simulink model "GATE_B"  (R2016a)
settings: Solver=FixedStepDiscrete  StartTime=0.0  StopTime=10.0  FixedStep=0.001  RelTol=1e-3
values from neighbouring files (symbols this model uses):
  CLOSE_CHAR = CHAR_STAR    [GateParameter.m]
  CLOSE_SIDE_VALUE = single(4*ONE_SEC)    [GateParameter.m]
  CLOSED = uint8(12)    [GateParameter.m]
  CLOSING = uint8(13)    [GateParameter.m]
  CURRENT_STABLE_TIMER = uint8(200)    [GateParameter.m]
  CURRENT_THRESH = uint16(1000)    [GateParameter.m]
  INIT = uint8(15)    [GateParameter.m]
  MOVING_TIMER = uint32(60*ONE_SEC)    [GateParameter.m]
  NO_PASS_ASSIG = uint8(6)    [GateParameter.m]
  OPEN = uint8(14)    [GateParameter.m]
  OPEN_CHAR = CHAR_HASH    [GateParameter.m]
  OPEN_SIDE_VALUE = uint16(4*ONE_SEC)    [GateParameter.m]
  OPENING = uint8(11)    [GateParameter.m]
  OPENING_ACTIVE = uint8(1)    [GateParameter.m]
  PASS_ASSIGNED = uint8(7)    [GateParameter.m]
  PASS_INCOMPLETE = uint8(8)    [GateParameter.m]
  PASS_TIMEOUT = uint16(10*ONE_SEC)    [GateParameter.m]
  PASSWORD_VERIFIED = uint8(5)    [GateParameter.m]
  STABLE_TIMER_VALUE = uint16(1*ONE_SEC)    [GateParameter.m]
  TIMEOUT = uint8(9)    [GateParameter.m]
  WRONG_PASSWORD = uint8(2)    [GateParameter.m]
settings Model: ExtModeTrigDuration=2  Creator=omaro  LastModifiedBy=oelkawok
settings OptimizationCC: DefaultParameterBehavior=Inlined  OptimizeModelRefInitCode=on  LifeSpan=1
settings HardwareCC: ProdLongLongMode=on
settings RTWCC: SystemTargetFile=ert.tlc  TemplateMakefile=ert_default_tmf  GenerateReport=on  IncludeHyperlinkInReport=on  LaunchReport=on  PortableWordSizes=on  GenerateTraceInfo=on  GenerateTraceReport=on  GenerateTraceReportSl=on  GenerateTraceReportSf=on  GenerateTraceReportEml=on
settings CodeAppCC: ForceParamTrailComments=on  IgnoreCustomStorageClasses=off  OperatorAnnotations=on  SimulinkDataObjDesc=on  SFDataObjDesc=on  MATLABFcnDesc=on  InsertBlockDesc=on  MATLABSourceComments=on
settings ERTTargetCC: GenerateSampleERTMain=on  InlinedParameterPlacement=NonHierarchical  ERTCustomFileTemplate=example_file_process.tlc

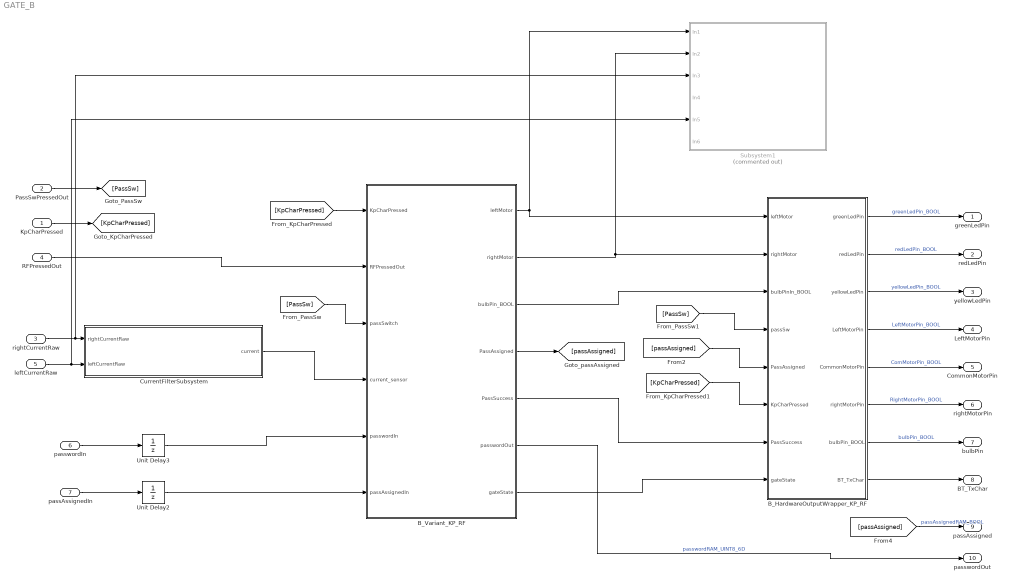
== system GATE_B ==
  KpCharPressed : Inport  OutDataTypeStr=uint8
  PassSwPressedOut : Inport  Port=2  OutDataTypeStr=boolean
  rightCurrentRaw : Inport  Port=3  OutDataTypeStr=uint16
  RFPressedOut : Inport  Port=4  OutDataTypeStr=uint8
  leftCurrentRaw : Inport  Port=5  OutDataTypeStr=uint16
  passwordIn : Inport  Port=6  OutDataTypeStr=uint8  PortDimensions=6
  passAssignedIn : Inport  Port=7  OutDataTypeStr=boolean
  B_HardwareOutputWrapper_KP_RF : Subsystem  VariantControl=Variant2
  B_Variant_KP_RF : Subsystem  VariantControl=Variant2
  CurrentFilterSubsystem : Subsystem
  Subsystem1 : Subsystem  Commented=on
  Unit Delay2 : UnitDelay  SampleTime=-1
  Unit Delay3 : UnitDelay  SampleTime=-1
  greenLedPin : Outport  OutDataTypeStr=boolean  PortDimensions=1  SampleTime=[0.001,0]
  redLedPin : Outport  Port=2  OutDataTypeStr=boolean  PortDimensions=1  SampleTime=[0.001,0]
  yellowLedPin : Outport  Port=3  OutDataTypeStr=boolean  PortDimensions=1  SampleTime=[0.001,0]
  LeftMotorPin : Outport  Port=4  OutDataTypeStr=boolean  PortDimensions=1  SampleTime=[0.001,0]
  CommonMotorPin : Outport  Port=5  OutDataTypeStr=boolean  PortDimensions=1  SampleTime=[0.001,0]
  rightMotorPin : Outport  Port=6  OutDataTypeStr=boolean  PortDimensions=1  SampleTime=[0.001,0]
  bulbPin : Outport  Port=7  OutDataTypeStr=boolean  PortDimensions=1  SampleTime=[0.001,0]
  BT_TxChar : Outport  Port=8  OutDataTypeStr=double  PortDimensions=1  SampleTime=[0.001,0]
  passAssigned : Outport  Port=9  OutDataTypeStr=boolean  PortDimensions=1  SampleTime=[0.001,0]
  passwordOut : Outport  Port=10  OutDataTypeStr=uint8  PortDimensions=6  SampleTime=[0.001,0]
  wires:
  CurrentFilterSubsystem/1(current) -> B_Variant_KP_RF/4(current_sensor)
  B_Variant_KP_RF/5(PassSuccess) -> B_HardwareOutputWrapper_KP_RF/7(PassSuccess)
  Unit Delay3/1 -> B_Variant_KP_RF/5(passwordIn)
  Unit Delay2/1 -> B_Variant_KP_RF/6(passAssignedIn)
  B_Variant_KP_RF/6(passwordOut) -> passwordOut/1  "passwordRAM_UINT8_6D"
  [passAssigned] -> B_HardwareOutputWrapper_KP_RF/5(PassAssigned)
  B_Variant_KP_RF/4(PassAssigned) -> [passAssigned]
  B_HardwareOutputWrapper_KP_RF/8(BT_TxChar) -> BT_TxChar/1
  B_HardwareOutputWrapper_KP_RF/7(bulbPin_BOOL) -> bulbPin/1  "bulbPin_BOOL"
  B_HardwareOutputWrapper_KP_RF/6(rightMotorPin) -> rightMotorPin/1  "RightMotorPin_BOOL"
  B_HardwareOutputWrapper_KP_RF/5(CommonMotorPin) -> CommonMotorPin/1  "ComMotorPin_BOOL"
  B_HardwareOutputWrapper_KP_RF/4(LeftMotorPin) -> LeftMotorPin/1  "LeftMotorPin_BOOL"
  B_HardwareOutputWrapper_KP_RF/3(yellowLedPin) -> yellowLedPin/1  "yellowLedPin_BOOL"
  B_HardwareOutputWrapper_KP_RF/2(redLedPin) -> redLedPin/1  "redLedPin_BOOL"
  B_HardwareOutputWrapper_KP_RF/1(greenLedPin) -> greenLedPin/1  "greenLedPin_BOOL"
  [KpCharPressed] -> B_HardwareOutputWrapper_KP_RF/6(KpCharPressed)
  [PassSw] -> B_HardwareOutputWrapper_KP_RF/4(passSw)
  B_Variant_KP_RF/3(bulbPin_BOOL) -> B_HardwareOutputWrapper_KP_RF/3(bulbPinIn_BOOL)
  B_Variant_KP_RF/1(leftMotor) -> B_HardwareOutputWrapper_KP_RF/1(leftMotor), Subsystem1/1(In1)
  [KpCharPressed] -> B_Variant_KP_RF/1(KpCharPressed)
  rightCurrentRaw/1 -> CurrentFilterSubsystem/1(rightCurrentRaw), Subsystem1/3(In3)
  [PassSw] -> B_Variant_KP_RF/3(passSwitch)
  RFPressedOut/1 -> B_Variant_KP_RF/2(RFPressedOut)
  KpCharPressed/1 -> [KpCharPressed]
  PassSwPressedOut/1 -> [PassSw]
  leftCurrentRaw/1 -> CurrentFilterSubsystem/2(leftCurrentRaw), Subsystem1/5(In5)
  [passAssigned] -> passAssigned/1  "passAssignedRAM_BOOL"
  passAssignedIn/1 -> Unit Delay2/1
  passwordIn/1 -> Unit Delay3/1
  B_Variant_KP_RF/2(rightMotor) -> B_HardwareOutputWrapper_KP_RF/2(rightMotor), Subsystem1/2(In2)
  B_Variant_KP_RF/7(gateState) -> B_HardwareOutputWrapper_KP_RF/8(gateState)

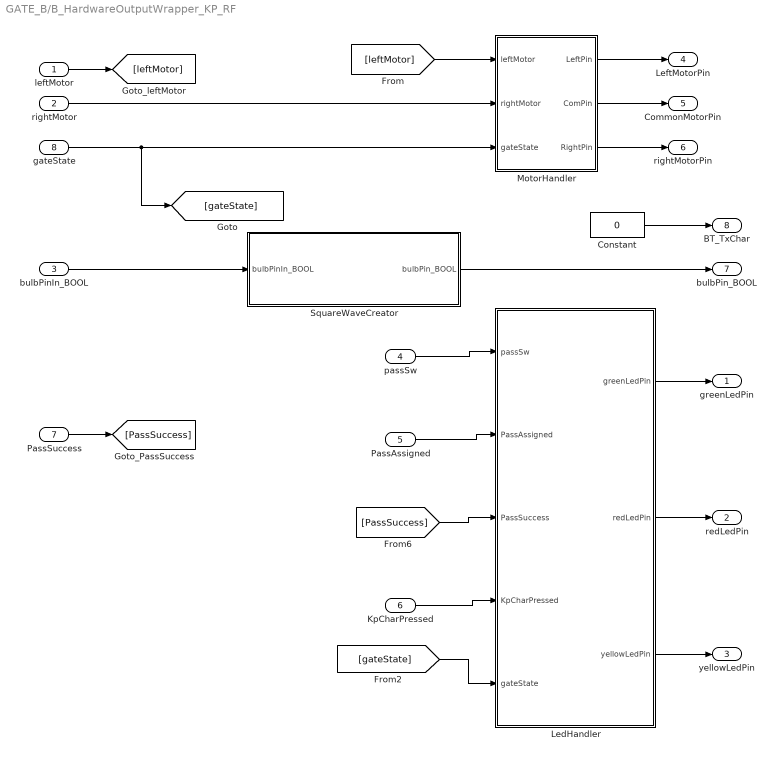
== system GATE_B/B_HardwareOutputWrapper_KP_RF ==
  leftMotor : Inport
  rightMotor : Inport  Port=2
  bulbPinIn_BOOL : Inport  Port=3
  passSw : Inport  Port=4
  PassAssigned : Inport  Port=5
  KpCharPressed : Inport  Port=6
  PassSuccess : Inport  Port=7
  gateState : Inport  Port=8
  Constant : Constant  Value=0  SampleTime=-1
  LedHandler : Subsystem
  MotorHandler : Subsystem
  SquareWaveCreator : Subsystem
  greenLedPin : Outport
  redLedPin : Outport  Port=2
  yellowLedPin : Outport  Port=3
  LeftMotorPin : Outport  Port=4
  CommonMotorPin : Outport  Port=5
  rightMotorPin : Outport  Port=6
  bulbPin_BOOL : Outport  Port=7
  BT_TxChar : Outport  Port=8
  wires:
  [gateState] -> LedHandler/5(gateState)
  SquareWaveCreator/1(bulbPin_BOOL) -> bulbPin_BOOL/1
  gateState/1 -> MotorHandler/3(gateState), [gateState]
  Constant/1 -> BT_TxChar/1
  PassSuccess/1 -> [PassSuccess]
  KpCharPressed/1 -> LedHandler/4(KpCharPressed)
  [PassSuccess] -> LedHandler/3(PassSuccess)
  PassAssigned/1 -> LedHandler/2(PassAssigned)
  passSw/1 -> LedHandler/1(passSw)
  leftMotor/1 -> [leftMotor]
  bulbPinIn_BOOL/1 -> SquareWaveCreator/1(bulbPinIn_BOOL)
  MotorHandler/3(RightPin) -> rightMotorPin/1
  MotorHandler/2(ComPin) -> CommonMotorPin/1
  MotorHandler/1(LeftPin) -> LeftMotorPin/1
  LedHandler/3(yellowLedPin) -> yellowLedPin/1
  LedHandler/2(redLedPin) -> redLedPin/1
  LedHandler/1(greenLedPin) -> greenLedPin/1
  [leftMotor] -> MotorHandler/1(leftMotor)
  rightMotor/1 -> MotorHandler/2(rightMotor)

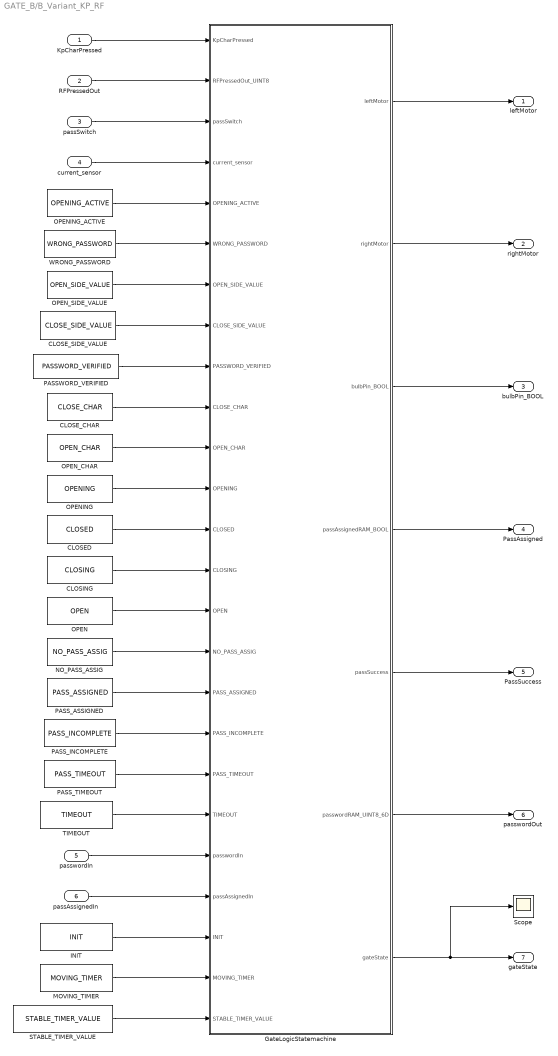
== system GATE_B/B_Variant_KP_RF ==
  KpCharPressed : Inport
  RFPressedOut : Inport  Port=2
  passSwitch : Inport  Port=3
  current_sensor : Inport  Port=4
  passwordIn : Inport  Port=5
  passAssignedIn : Inport  Port=6
  CLOSED : Constant  Value=CLOSED  SampleTime=-1
  CLOSE_CHAR : Constant  Value=CLOSE_CHAR  SampleTime=-1
  CLOSE_SIDE_VALUE : Constant  Value=CLOSE_SIDE_VALUE  SampleTime=-1
  CLOSING : Constant  Value=CLOSING  SampleTime=-1
  GateLogicStatemachine : Stateflow chart  TreatAsAtomicUnit=on
  INIT : Constant  Value=INIT  SampleTime=-1
  MOVING_TIMER : Constant  Value=MOVING_TIMER  SampleTime=-1
  NO_PASS_ASSIG : Constant  Value=NO_PASS_ASSIG  SampleTime=-1
  OPEN : Constant  Value=OPEN  SampleTime=-1
  OPENING : Constant  Value=OPENING  SampleTime=-1
  OPENING_ACTIVE : Constant  Value=OPENING_ACTIVE  SampleTime=-1
  OPEN_CHAR : Constant  Value=OPEN_CHAR  SampleTime=-1
  OPEN_SIDE_VALUE : Constant  Value=OPEN_SIDE_VALUE  SampleTime=-1
  PASSWORD_VERIFIED : Constant  Value=PASSWORD_VERIFIED  SampleTime=-1
  PASS_ASSIGNED : Constant  Value=PASS_ASSIGNED  SampleTime=-1
  PASS_INCOMPLETE : Constant  Value=PASS_INCOMPLETE  SampleTime=-1
  PASS_TIMEOUT : Constant  Value=PASS_TIMEOUT  SampleTime=-1
  STABLE_TIMER_VALUE : Constant  Value=STABLE_TIMER_VALUE  SampleTime=-1
  Scope : Scope
  TIMEOUT : Constant  Value=TIMEOUT  SampleTime=-1
  WRONG_PASSWORD : Constant  Value=WRONG_PASSWORD  SampleTime=-1
  leftMotor : Outport
  rightMotor : Outport  Port=2
  bulbPin_BOOL : Outport  Port=3
  PassAssigned : Outport  Port=4
  PassSuccess : Outport  Port=5
  passwordOut : Outport  Port=6
  gateState : Outport  Port=7
  wires:
  STABLE_TIMER_VALUE/1 -> GateLogicStatemachine/25(STABLE_TIMER_VALUE)
  MOVING_TIMER/1 -> GateLogicStatemachine/24(MOVING_TIMER)
  INIT/1 -> GateLogicStatemachine/23(INIT)
  GateLogicStatemachine/7(gateState) -> gateState/1, Scope/1
  CLOSING/1 -> GateLogicStatemachine/14(CLOSING)
  OPENING/1 -> GateLogicStatemachine/12(OPENING)
  CLOSED/1 -> GateLogicStatemachine/13(CLOSED)
  OPEN_CHAR/1 -> GateLogicStatemachine/11(OPEN_CHAR)
  CLOSE_CHAR/1 -> GateLogicStatemachine/10(CLOSE_CHAR)
  OPEN/1 -> GateLogicStatemachine/15(OPEN)
  PASSWORD_VERIFIED/1 -> GateLogicStatemachine/9(PASSWORD_VERIFIED)
  RFPressedOut/1 -> GateLogicStatemachine/2(RFPressedOut_UINT8)
  GateLogicStatemachine/3(bulbPin_BOOL) -> bulbPin_BOOL/1
  current_sensor/1 -> GateLogicStatemachine/4(current_sensor)
  WRONG_PASSWORD/1 -> GateLogicStatemachine/6(WRONG_PASSWORD)
  GateLogicStatemachine/1(leftMotor) -> leftMotor/1
  GateLogicStatemachine/2(rightMotor) -> rightMotor/1
  OPENING_ACTIVE/1 -> GateLogicStatemachine/5(OPENING_ACTIVE)
  OPEN_SIDE_VALUE/1 -> GateLogicStatemachine/7(OPEN_SIDE_VALUE)
  CLOSE_SIDE_VALUE/1 -> GateLogicStatemachine/8(CLOSE_SIDE_VALUE)
  NO_PASS_ASSIG/1 -> GateLogicStatemachine/16(NO_PASS_ASSIG)
  KpCharPressed/1 -> GateLogicStatemachine/1(KpCharPressed)
  PASS_TIMEOUT/1 -> GateLogicStatemachine/19(PASS_TIMEOUT)
  GateLogicStatemachine/5(passSuccess) -> PassSuccess/1
  passSwitch/1 -> GateLogicStatemachine/3(passSwitch)
  GateLogicStatemachine/4(passAssignedRAM_BOOL) -> PassAssigned/1
  PASS_ASSIGNED/1 -> GateLogicStatemachine/17(PASS_ASSIGNED)
  PASS_INCOMPLETE/1 -> GateLogicStatemachine/18(PASS_INCOMPLETE)
  TIMEOUT/1 -> GateLogicStatemachine/20(TIMEOUT)
  passwordIn/1 -> GateLogicStatemachine/21(passwordIn)
  passAssignedIn/1 -> GateLogicStatemachine/22(passAssignedIn)
  GateLogicStatemachine/6(passwordRAM_UINT8_6D) -> passwordOut/1

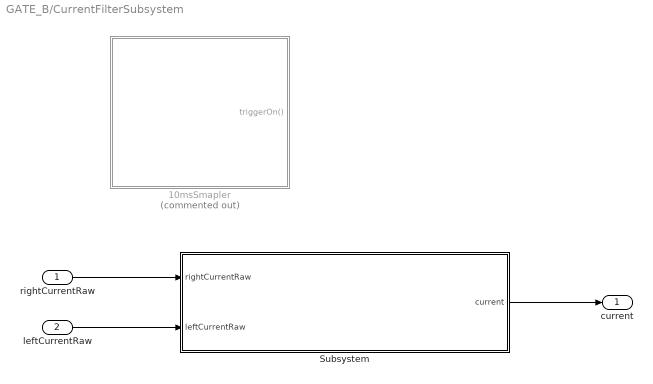
== system GATE_B/CurrentFilterSubsystem ==
  rightCurrentRaw : Inport
  leftCurrentRaw : Inport  Port=2
  10msSmapler : Stateflow chart  Commented=on  TreatAsAtomicUnit=on
  Subsystem : Subsystem
  current : Outport
  wires:
  leftCurrentRaw/1 -> Subsystem/2(leftCurrentRaw)
  rightCurrentRaw/1 -> Subsystem/1(rightCurrentRaw)
  Subsystem/1(current) -> current/1

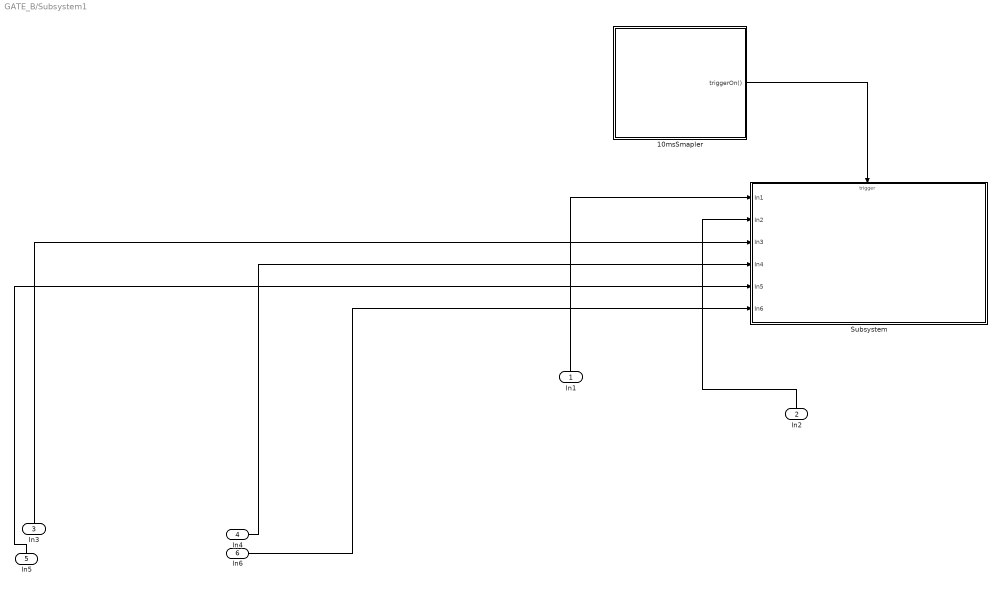
== system GATE_B/Subsystem1 ==
  In1 : Inport
  In2 : Inport  Port=2
  In3 : Inport  Port=3
  In4 : Inport  Port=4
  In5 : Inport  Port=5
  In6 : Inport  Port=6
  10msSmapler : Stateflow chart  TreatAsAtomicUnit=on
  Subsystem : Subsystem
  wires:
  In4/1 -> Subsystem/4(In4)
  10msSmapler/1(triggerOn()) -> Subsystem/Trigger
  In6/1 -> Subsystem/6(In6)
  In5/1 -> Subsystem/5(In5)
  In2/1 -> Subsystem/2(In2)
  In1/1 -> Subsystem/1(In1)
  In3/1 -> Subsystem/3(In3)

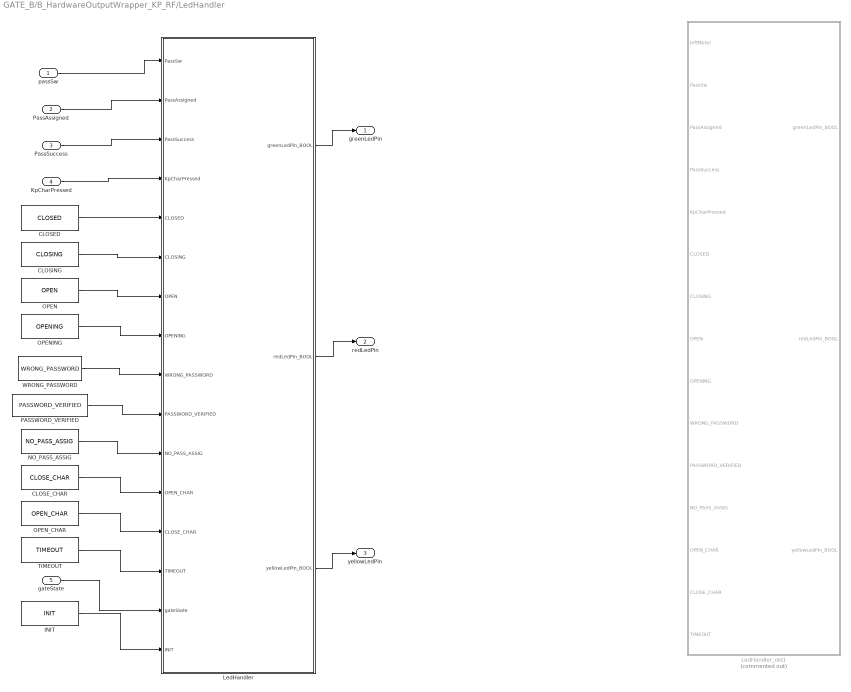
== system GATE_B/B_HardwareOutputWrapper_KP_RF/LedHandler ==
  passSw : Inport
  PassAssigned : Inport  Port=2
  PassSuccess : Inport  Port=3
  KpCharPressed : Inport  Port=4
  gateState : Inport  Port=5
  CLOSED : Constant  Value=CLOSED  SampleTime=-1
  CLOSE_CHAR : Constant  Value=CLOSE_CHAR  SampleTime=-1
  CLOSING : Constant  Value=CLOSING  SampleTime=-1
  INIT : Constant  Value=INIT  SampleTime=-1
  LedHandler : Stateflow chart  TreatAsAtomicUnit=on
  LedHandler_old1 : Stateflow chart  Commented=on  TreatAsAtomicUnit=on
  NO_PASS_ASSIG : Constant  Value=NO_PASS_ASSIG  SampleTime=-1
  OPEN : Constant  Value=OPEN  SampleTime=-1
  OPENING : Constant  Value=OPENING  SampleTime=-1
  OPEN_CHAR : Constant  Value=OPEN_CHAR  SampleTime=-1
  PASSWORD_VERIFIED : Constant  Value=PASSWORD_VERIFIED  SampleTime=-1
  TIMEOUT : Constant  Value=TIMEOUT  SampleTime=-1
  WRONG_PASSWORD : Constant  Value=WRONG_PASSWORD  SampleTime=-1
  greenLedPin : Outport
  redLedPin : Outport  Port=2
  yellowLedPin : Outport  Port=3
  wires:
  INIT/1 -> LedHandler/16(INIT)
  gateState/1 -> LedHandler/15(gateState)
  TIMEOUT/1 -> LedHandler/14(TIMEOUT)
  OPEN_CHAR/1 -> LedHandler/13(CLOSE_CHAR)
  CLOSE_CHAR/1 -> LedHandler/12(OPEN_CHAR)
  KpCharPressed/1 -> LedHandler/4(KpCharPressed)
  NO_PASS_ASSIG/1 -> LedHandler/11(NO_PASS_ASSIG)
  PASSWORD_VERIFIED/1 -> LedHandler/10(PASSWORD_VERIFIED)
  WRONG_PASSWORD/1 -> LedHandler/9(WRONG_PASSWORD)
  CLOSED/1 -> LedHandler/5(CLOSED)
  CLOSING/1 -> LedHandler/6(CLOSING)
  OPEN/1 -> LedHandler/7(OPEN)
  OPENING/1 -> LedHandler/8(OPENING)
  PassSuccess/1 -> LedHandler/3(PassSuccess)
  PassAssigned/1 -> LedHandler/2(PassAssigned)
  passSw/1 -> LedHandler/1(PassSw)
  LedHandler/3(yellowLedPin_BOOL) -> yellowLedPin/1
  LedHandler/2(redLedPin_BOOL) -> redLedPin/1
  LedHandler/1(greenLedPin_BOOL) -> greenLedPin/1

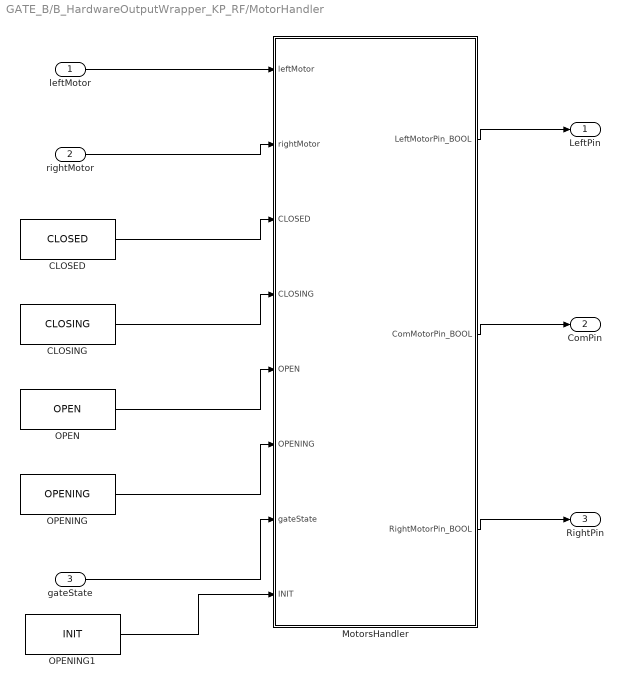
== system GATE_B/B_HardwareOutputWrapper_KP_RF/MotorHandler ==
  leftMotor : Inport
  rightMotor : Inport  Port=2
  gateState : Inport  Port=3
  CLOSED : Constant  Value=CLOSED  SampleTime=-1
  CLOSING : Constant  Value=CLOSING  SampleTime=-1
  MotorsHandler : Stateflow chart  TreatAsAtomicUnit=on
  OPEN : Constant  Value=OPEN  SampleTime=-1
  OPENING : Constant  Value=OPENING  SampleTime=-1
  OPENING1 : Constant  Value=INIT  SampleTime=-1
  LeftPin : Outport
  ComPin : Outport  Port=2
  RightPin : Outport  Port=3
  wires:
  OPENING1/1 -> MotorsHandler/8(INIT)
  leftMotor/1 -> MotorsHandler/1(leftMotor)
  gateState/1 -> MotorsHandler/7(gateState)
  MotorsHandler/3(RightMotorPin_BOOL) -> RightPin/1
  MotorsHandler/2(ComMotorPin_BOOL) -> ComPin/1
  MotorsHandler/1(LeftMotorPin_BOOL) -> LeftPin/1
  OPENING/1 -> MotorsHandler/6(OPENING)
  OPEN/1 -> MotorsHandler/5(OPEN)
  CLOSING/1 -> MotorsHandler/4(CLOSING)
  CLOSED/1 -> MotorsHandler/3(CLOSED)
  rightMotor/1 -> MotorsHandler/2(rightMotor)

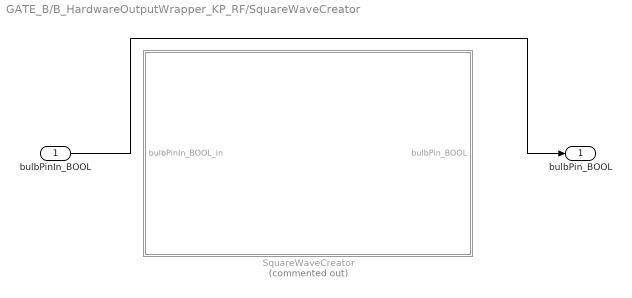
== system GATE_B/B_HardwareOutputWrapper_KP_RF/SquareWaveCreator ==
  bulbPinIn_BOOL : Inport
  SquareWaveCreator : Stateflow chart  Commented=on  TreatAsAtomicUnit=on
  bulbPin_BOOL : Outport
  wires:
  bulbPinIn_BOOL/1 -> bulbPin_BOOL/1

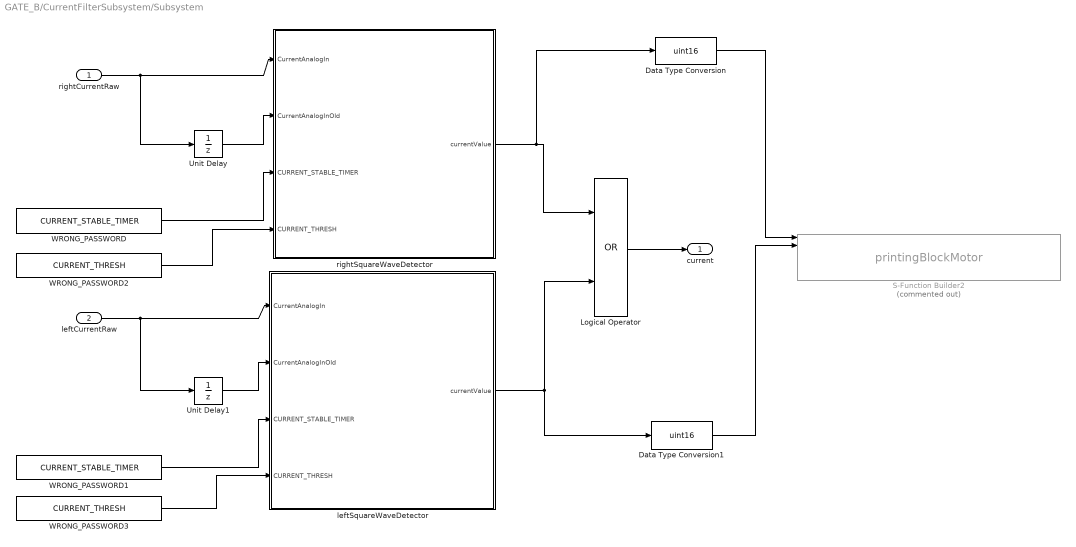
== system GATE_B/CurrentFilterSubsystem/Subsystem ==
  rightCurrentRaw : Inport
  leftCurrentRaw : Inport  Port=2
  Data Type Conversion : DataTypeConversion  OutDataTypeStr=uint16
  Data Type Conversion1 : DataTypeConversion  OutDataTypeStr=uint16
  Logical Operator : Logic  Operator=OR  AllPortsSameDT=off  OutDataTypeStr=boolean
  S-Function Builder2 : S-Function  Commented=on  InitFcn=try, set_param(gcb,'FunctionName','printingBlockMotor'), end  FunctionName=printingBlockMotor  SFunctionModules=printingBlockMotor_wrapper  SFunctionDeploymentMode=off  EnableBusSupport=off  mask(S-Function Builder){}
      mask help: Simulink:masks:SFunctionBuilder_MD
      mask init:
      | val = [[.9  0.75 0.75 1 1 .9 .9 1]',[1 1 0.75 0.75 .9 .9 1 .9]'];try , sys = get_param(gcb,'SfunBuilderFcnName');if isempty(sys), sys = get_param(gcb,'FunctionName'); end,catch, sys = get_param(gcb,'FunctionName'); end
      settings: CopyFcn=set_param(gcbh,'LinkStatus','none')  PreSaveFcn=try, set_param(gcb,'FunctionName','printingBlockMotor'), end  OpenFcn=sfunctionwizard(gcbh)
      mask Display: plot(val(:,1),val(:,2)),disp(sys), port_label('input',1,'u0'), port_label('input',2,'u1')
  Unit Delay : UnitDelay  SampleTime=-1
  Unit Delay1 : UnitDelay  SampleTime=-1
  WRONG_PASSWORD : Constant  Value=CURRENT_STABLE_TIMER  SampleTime=-1
  WRONG_PASSWORD1 : Constant  Value=CURRENT_STABLE_TIMER  SampleTime=-1
  WRONG_PASSWORD2 : Constant  Value=CURRENT_THRESH  SampleTime=-1
  WRONG_PASSWORD3 : Constant  Value=CURRENT_THRESH  SampleTime=-1
  leftSquareWaveDetector : Stateflow chart  TreatAsAtomicUnit=on
  rightSquareWaveDetector : Stateflow chart  TreatAsAtomicUnit=on
  current : Outport
  wires:
  WRONG_PASSWORD3/1 -> leftSquareWaveDetector/4(CURRENT_THRESH)
  WRONG_PASSWORD2/1 -> rightSquareWaveDetector/4(CURRENT_THRESH)
  WRONG_PASSWORD1/1 -> leftSquareWaveDetector/3(CURRENT_STABLE_TIMER)
  WRONG_PASSWORD/1 -> rightSquareWaveDetector/3(CURRENT_STABLE_TIMER)
  Data Type Conversion1/1 -> S-Function Builder2/2
  Data Type Conversion/1 -> S-Function Builder2/1
  Logical Operator/1 -> current/1
  leftSquareWaveDetector/1(currentValue) -> Data Type Conversion1/1, Logical Operator/2
  rightSquareWaveDetector/1(currentValue) -> Logical Operator/1, Data Type Conversion/1
  Unit Delay1/1 -> leftSquareWaveDetector/2(CurrentAnalogInOld)
  leftCurrentRaw/1 -> leftSquareWaveDetector/1(CurrentAnalogIn), Unit Delay1/1
  Unit Delay/1 -> rightSquareWaveDetector/2(CurrentAnalogInOld)
  rightCurrentRaw/1 -> Unit Delay/1, rightSquareWaveDetector/1(CurrentAnalogIn)

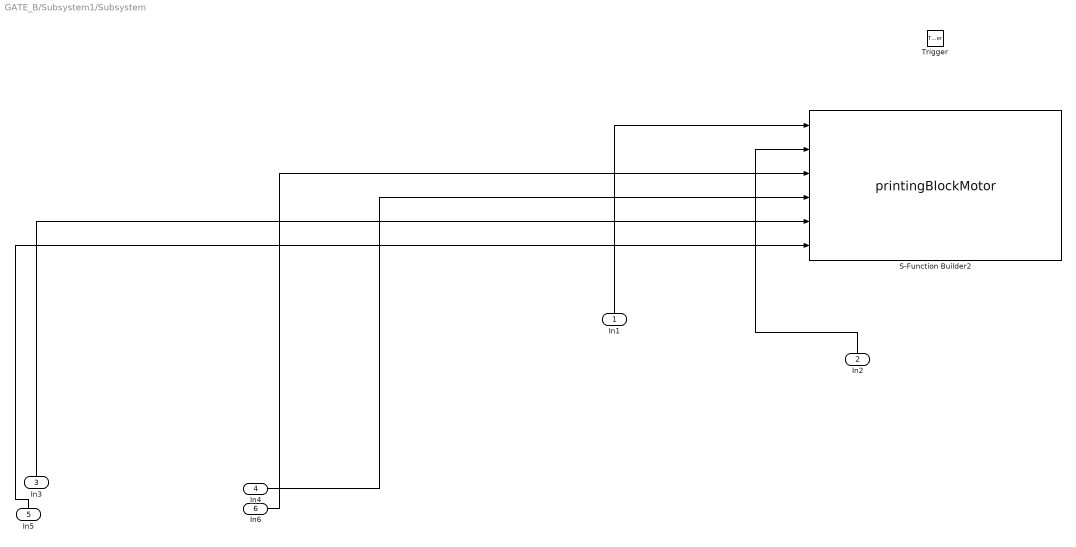
== system GATE_B/Subsystem1/Subsystem ==
  In1 : Inport
  In2 : Inport  Port=2
  In3 : Inport  Port=3
  In4 : Inport  Port=4
  In5 : Inport  Port=5
  In6 : Inport  Port=6
  Trigger : TriggerPort  TriggerType=function-call  VariantControl=Variant  PortDimensions=1
  S-Function Builder2 : S-Function  InitFcn=try, set_param(gcb,'FunctionName','printingBlockMotor'), end  FunctionName=printingBlockMotor  SFunctionModules=printingBlockMotor_wrapper  SFunctionDeploymentMode=off  EnableBusSupport=off  mask(S-Function Builder){}
      mask help: Simulink:masks:SFunctionBuilder_MD
      mask init: same as GATE_B/CurrentFilterSubsystem/Subsystem/S-Function Builder2
      settings: CopyFcn=set_param(gcbh,'LinkStatus','none')  PreSaveFcn=try, set_param(gcb,'FunctionName','printingBlockMotor'), end  OpenFcn=sfunctionwizard(gcbh)
      mask Display: plot(val(:,1),val(:,2)),disp(sys), port_label('input',1,'leftMotor'), port_label('input',2,'rightMotor'), port_label('input',3,'leftCurr'), port_label('input',4,'rightCurr'), port_label('input',5,'rightCurrRaw'), port_label('input',6,'leftCurrRaw')
  wires:
  In2/1 -> S-Function Builder2/2
  In1/1 -> S-Function Builder2/1
  In3/1 -> S-Function Builder2/5
  In5/1 -> S-Function Builder2/6
  In4/1 -> S-Function Builder2/4
  In6/1 -> S-Function Builder2/3

== stateflow chart GATE_B/CurrentFilterSubsystem/Subsystem/leftSquareWaveDetector ==
  state Running
    entry:
    counterHigh = 0;
    counterLow= 0;
    currentValue = 1;
    state High
      entry:
      counterLow = 0;
    state Low
      entry:
      counterHigh = 0;
    (default) -> High
    High -> High [order 2] : [CurrentAnalogIn > CURRENT_THRESH]
        | /counterHigh++;
    High -> Low [order 1] : [CurrentAnalogIn < CURRENT_THRESH]
    Low -> High [order 1] : [CurrentAnalogIn > CURRENT_THRESH]
    Low -> Low [order 2] : [CurrentAnalogIn < CURRENT_THRESH]
        | /counterLow++;
  state Stop
    entry:
    currentValue = 0;
    stableCounter = 0;
  (default) -> Stop
  Stop -> Running : [((CurrentAnalogInOld > CURRENT_THRESH)...
      |  && (CurrentAnalogIn < CURRENT_THRESH)) ...
      | || ((CurrentAnalogInOld < CURRENT_THRESH)...
      |  && (CurrentAnalogIn > CURRENT_THRESH))]
  Running -> Stop : [(counterHigh >= CURRENT_STABLE_TIMER)...
      |  || (counterLow >= CURRENT_STABLE_TIMER)]
  data: CurrentAnalogIn input; currentValue output uint8; counterHigh local uint16; counterLow local uint16; stableCounter local uint8; CurrentAnalogInOld input; CURRENT_STABLE_TIMER input; CURRENT_THRESH input

== stateflow chart GATE_B/Subsystem1/10msSmapler ==
  (default) -> (junction 2)
  (junction 2) -> (junction 3) : {counter_1ms++;}
  (junction 3) -> (junction 6) : [counter_1ms == 10]
      | {
      | triggerOn;
      | counter_1ms = 0;
      | }
  data: counter_1ms local double
  events: triggerOn output FUNCTION_CALL_EVENT

== stateflow chart GATE_B/B_HardwareOutputWrapper_KP_RF/SquareWaveCreator/SquareWaveCreator ==
  state BulbOn
    state Off
      entry:
      counter = 0;
      bulbPin_BOOL = false;
      du:
      counter++;
    state On
      entry:
      counter = 0;
      bulbPin_BOOL = true;
      du:
      counter++;
    (default) -> Off
    On -> Off : [counter >= 1000]/counter = 0;
    Off -> On : [counter >= 1000]/counter = 0;
  state BulbOff
    entry:
    bulbPin_BOOL = false;
  (default) -> BulbOff
  BulbOff -> BulbOn : [bulbPinIn_BOOL_in]
  BulbOn -> BulbOff : [!bulbPinIn_BOOL_in]
  data: bulbPinIn_BOOL_in input; bulbPin_BOOL output boolean; counter local uint16

== stateflow chart GATE_B/B_HardwareOutputWrapper_KP_RF/LedHandler/LedHandler_old1 ==
  state AssigningPass
    en:
    counter = 0;
    state Start
      en:
      yellowLedPin_BOOL = true;
      greenLedPin_BOOL = false;
      redLedPin_BOOL = false;
    state correctPassAssigned
      du:
      counter++;
    state incorrectPassAssigned
      du:
      counter++;
    (default) -> AssigningPass.Start
    AssigningPass.Start -> correctPassAssigned [order 1] : [PassAssigned == true]/greenLedPin_BOOL = true;
    AssigningPass.Start -> incorrectPassAssigned [order 2] : [(PassSw == false) && (PassAssigned == false)]
        | /redLedPin_BOOL = true;...
        | yellowLedPin_BOOL = false;
    correctPassAssigned -> correctPassAssigned : [(hasChanged(PassSw)) ...
        | && (PassSw == false)]
        | /yellowLedPin_BOOL = false;
  state EnteringPass
    en:
    counter = 0;
    state correctPass
      en:
      yellowLedPin_BOOL = false;
      greenLedPin_BOOL = true;
      redLedPin_BOOL = false;
      du:
      counter++;
    state Start
    state IncorrectPass
      en:
      yellowLedPin_BOOL = false;
      greenLedPin_BOOL = false;
      redLedPin_BOOL = true;
      du:
      counter++;
    EnteringPass.Start -> correctPass [order 1] : [PassSuccess == PASSWORD_VERIFIED]
    (default) -> EnteringPass.Start
    EnteringPass.Start -> IncorrectPass [order 2] : [(PassSuccess == TIMEOUT)...
        |  || (PassSuccess == WRONG_PASSWORD)]
  state Idle
    en:
    yellowLedPin_BOOL = false;
    greenLedPin_BOOL = false;
    redLedPin_BOOL = false;
  state GateOn
    en:
    yellowLedPin_BOOL = false;
    greenLedPin_BOOL = true;
    redLedPin_BOOL = false;
  (default) -> Idle
  EnteringPass -> Idle [order 2] : [PassSuccess == NO_PASS_ASSIG]
  Idle -> AssigningPass [order 1] : [PassSw == true]
  correctPass -> Idle : [counter >= 4800]
  AssigningPass -> Idle [order 1] : [(counter >= 4900)]
  Idle -> EnteringPass [order 2] : [(hasChanged(KpCharPressed)) ...
      | && (KpCharPressed != 0)...
      | && (KpCharPressed != OPEN_CHAR)...
      | && (KpCharPressed != CLOSE_CHAR)...
      | && (PassAssigned == true)]
      | /yellowLedPin_BOOL = true;
  IncorrectPass -> Idle : [counter >= 4800]
  Idle -> GateOn [order 3] : [(leftMotor == OPENING)...
      |  || (leftMotor == OPEN)...
      |  || (leftMotor == CLOSING)]
  GateOn -> Idle : [leftMotor == CLOSED]
  EnteringPass -> GateOn [order 1] : [(leftMotor == OPENING)...
      | || (leftMotor == OPEN)...
      | || (leftMotor == CLOSING)]
  AssigningPass -> GateOn [order 2] : [(leftMotor == OPENING)...
      |  || (leftMotor == OPEN)...
      |  || (leftMotor == CLOSING)]
  data: leftMotor input; greenLedPin_BOOL output boolean =false; redLedPin_BOOL output boolean =false; yellowLedPin_BOOL output boolean =false; PassSw input; counter local uint16; PassAssigned input; PassSuccess input; KpCharPressed input; CLOSED input; CLOSING input; OPEN input; OPENING input; WRONG_PASSWORD input; PASSWORD_VERIFIED input; NO_PASS_ASSIG input; OPEN_CHAR input; CLOSE_CHAR input; TIMEOUT input

== stateflow chart GATE_B/B_HardwareOutputWrapper_KP_RF/LedHandler/LedHandler ==
  state AssigningPass
    state Start
      en:
      counter = 0;
      yellowLedPin_BOOL = true;
      greenLedPin_BOOL = false;
      redLedPin_BOOL = false;
    state correctPassAssigned
      du:
      counter++;
    state incorrectPassAssigned
      du:
      counter++;
    (default) -> AssigningPass.Start
    AssigningPass.Start -> incorrectPassAssigned [order 2] : [(PassSw == false) && (PassAssigned == false)]
        | /redLedPin_BOOL = true;...
        | yellowLedPin_BOOL = false;
    AssigningPass.Start -> correctPassAssigned [order 1] : [PassAssigned == true]/greenLedPin_BOOL = true;
    correctPassAssigned -> correctPassAssigned : [(hasChanged(PassSw)) ...
        | && (PassSw == false)]
        | /yellowLedPin_BOOL = false;
  state EnteringPass
    en:
    counter = 0;
    state correctPass
      en:
      yellowLedPin_BOOL = false;
      greenLedPin_BOOL = true;
      redLedPin_BOOL = false;
      du:
      counter++;
    state Start
    state IncorrectPass
      en:
      yellowLedPin_BOOL = false;
      greenLedPin_BOOL = false;
      redLedPin_BOOL = true;
      du:
      counter++;
    EnteringPass.Start -> correctPass [order 1] : [PassSuccess == PASSWORD_VERIFIED]
    (default) -> EnteringPass.Start
    EnteringPass.Start -> IncorrectPass [order 2] : [(PassSuccess == TIMEOUT)...
        |  || (PassSuccess == WRONG_PASSWORD)]
  state Idle
    en:
    counter = 0;
    yellowLedPin_BOOL = false;
    greenLedPin_BOOL = false;
    redLedPin_BOOL = false;
  state GateOn
    en:
    yellowLedPin_BOOL = false;
    greenLedPin_BOOL = true;
    redLedPin_BOOL = false;
  (default) -> Idle
  EnteringPass -> Idle [order 2] : [PassSuccess == NO_PASS_ASSIG]
  Idle -> AssigningPass [order 1] : [PassSw == true]
  correctPass -> (junction 113)
  AssigningPass -> Idle [order 1] : [(counter >= 4900)]
  Idle -> (junction 113) [order 3]
  (junction 113) -> Idle [order 1] : [counter >= 4800]
  Idle -> GateOn [order 2] : [(gateState == OPENING)...
      |  || (gateState == OPEN)...
      |  || (gateState == CLOSING)]
  GateOn -> Idle : [gateState == CLOSED]
  (junction 113) -> EnteringPass [order 2] : [(hasChanged(KpCharPressed)) ...
      | && (KpCharPressed != 0)...
      | && (KpCharPressed != OPEN_CHAR)...
      | && (KpCharPressed != CLOSE_CHAR)...
      | && (PassAssigned == true)...
      | && (gateState != INIT)]
      | /yellowLedPin_BOOL = true;
      | greenLedPin_BOOL = false;
      | redLedPin_BOOL = false;
  IncorrectPass -> (junction 113)
  EnteringPass -> GateOn [order 1] : [(gateState == OPENING)...
      | || (gateState == OPEN)...
      | || (gateState == CLOSING)]
  AssigningPass -> GateOn [order 2] : [(gateState == OPENING)...
      |  || (gateState == OPEN)...
      |  || (gateState == CLOSING)]
  AssigningPass -> AssigningPass [order 3] : [hasChanged(PassSw) ...
      | && PassSw == true]
  data: greenLedPin_BOOL output boolean =false; redLedPin_BOOL output boolean =false; yellowLedPin_BOOL output boolean =false; PassSw input; counter local uint16; PassAssigned input; PassSuccess input; KpCharPressed input; CLOSED input; CLOSING input; OPEN input; OPENING input; WRONG_PASSWORD input; PASSWORD_VERIFIED input; NO_PASS_ASSIG input; OPEN_CHAR input; CLOSE_CHAR input; TIMEOUT input; gateState input; INIT input

== stateflow chart GATE_B/B_HardwareOutputWrapper_KP_RF/MotorHandler/MotorsHandler ==
  state MonitorChange
  state UpdatePins
    (default) -> (junction 91) : /* updating motor Pins Switch case */
    (junction 91) -> (junction 92) [order 1] : [(leftMotor == OPENING) && ((rightMotor == CLOSED) || (rightMotor == OPEN))]
    (junction 92) -> (junction 100) : {LeftMotorPin_BOOL = true;...
        | ComMotorPin_BOOL = true;...
        | RightMotorPin_BOOL = false;}
    (junction 91) -> (junction 93) [order 2]
    (junction 93) -> (junction 94) [order 1] : [(leftMotor == CLOSING) && ((rightMotor == CLOSED) || (rightMotor == OPEN))]
    (junction 94) -> (junction 99) : {LeftMotorPin_BOOL = false;...
        | ComMotorPin_BOOL = false;...
        |  RightMotorPin_BOOL = true;}
    (junction 93) -> (junction 95) [order 2]
    (junction 95) -> (junction 96) [order 1] : [(rightMotor == CLOSING) && ((leftMotor == CLOSED) || (leftMotor == OPEN))]
    (junction 96) -> (junction 98) : {LeftMotorPin_BOOL = true;...
        | ComMotorPin_BOOL = false;...
        | RightMotorPin_BOOL = false;}
    (junction 95) -> (junction 102) [order 2]
    (junction 102) -> (junction 103) [order 1] : [(rightMotor == OPENING) && ((leftMotor == CLOSED) || (leftMotor == OPEN))]
    (junction 103) -> (junction 110) : {LeftMotorPin_BOOL = false;...
        | ComMotorPin_BOOL = true;...
        | RightMotorPin_BOOL = true;}
    (junction 102) -> (junction 104) [order 2]
    (junction 104) -> (junction 105) [order 1] : [(rightMotor == OPENING) && (leftMotor == OPENING)]
    (junction 105) -> (junction 111) : {LeftMotorPin_BOOL = true;...
        | ComMotorPin_BOOL = true;...
        | RightMotorPin_BOOL = true;}
    (junction 104) -> (junction 106) [order 2]
    (junction 106) -> (junction 107) [order 1] : [(rightMotor == CLOSING) && (leftMotor == CLOSING)]
    (junction 106) -> (junction 123) [order 2]
    (junction 107) -> (junction 112) : {LeftMotorPin_BOOL = false;...
        | ComMotorPin_BOOL = false;...
        | RightMotorPin_BOOL = false;}
    (junction 123) -> (junction 124) [order 1] : [((rightMotor == CLOSED) || (rightMotor == OPEN)) ...
        | && ((leftMotor == CLOSED) || (leftMotor == OPEN))]
    (junction 123) -> (junction 136) [order 2]
    (junction 124) -> (junction 125) : {LeftMotorPin_BOOL = false;...
        | ComMotorPin_BOOL = true;...
        | RightMotorPin_BOOL = false;}
    (junction 136) -> (junction 138) [order 1] : [(gateState == CLOSED) || (gateState == OPEN) || (gateState == INIT)]
    (junction 136) -> (junction 97) [order 2]
    (junction 138) -> (junction 139) : {LeftMotorPin_BOOL = false;...
        | ComMotorPin_BOOL = true;...
        | RightMotorPin_BOOL = false;}
    (junction 100) -> (junction 99)
    (junction 99) -> (junction 98)
    (junction 98) -> (junction 110)
    (junction 139) -> (junction 97)
    (junction 125) -> (junction 139)
    (junction 112) -> (junction 125)
    (junction 111) -> (junction 112)
    (junction 110) -> (junction 111)
    (junction 97) -> (junction 101)
  (default) -> MonitorChange
  UpdatePins -> MonitorChange
  MonitorChange -> UpdatePins : [(hasChanged(leftMotor)) ...
      | || (hasChanged(rightMotor))...
      | || (hasChanged(gateState) && (gateState == CLOSED))...
      |  || (hasChanged(gateState) && (gateState == OPEN))...
      | ||(hasChanged(gateState) && (gateState == INIT))]
  data: leftMotor input; LeftMotorPin_BOOL output boolean =false; ComMotorPin_BOOL output boolean =true; RightMotorPin_BOOL output boolean =false; rightMotor input; CLOSED input; CLOSING input; OPEN input; OPENING input; gateState input; INIT input

== stateflow chart GATE_B/B_Variant_KP_RF/GateLogicStatemachine ==
  state init
    entry:
    passSuccess = NO_PASS_ASSIG;
    gotoReady = false;
    bulbPin_BOOL = 0;
    leftMotor = CLOSED;
    rightMotor = CLOSED;
    gateState = INIT;
    state AssignPass
      entry:
      counter = 0;
      passwordRAM_UINT8_6D[0] = 0;
      passwordRAM_UINT8_6D[1] = 0;
      passwordRAM_UINT8_6D[2] = 0;
      passwordRAM_UINT8_6D[3] = 0;
      passwordRAM_UINT8_6D[4] = 0;
      passwordRAM_UINT8_6D[5] = 0;
      state addToPass
        entry:
        passwordRAM_UINT8_6D[counter] = KpCharPressed;
      state MonitoringNumber
      state PassAssigned
        entry:
        gotoReady = true;
      MonitoringNumber -> (junction 259) [order 1] : [hasChanged(KpCharPressed)]
      (junction 259) -> addToPass : [KpCharPressed != 0]
      (default) -> MonitoringNumber
      addToPass -> MonitoringNumber [order 1] : [counter < 5]/counter++;
      MonitoringNumber -> PassAssigned [order 2] : [RFPressedOut_UINT8 == true]
      addToPass -> PassAssigned [order 2] : [counter == 5]
          | / passAssignedRAM_BOOL = true;...
          | passSuccess = PASS_ASSIGNED;
    state idle
      entry:
      passAssignedRAM_BOOL = false;
    state PassAssignedPreviously
      entry:
      passwordRAM_UINT8_6D[0] = passwordIn[0];
      passwordRAM_UINT8_6D[1] = passwordIn[1];
      passwordRAM_UINT8_6D[2] = passwordIn[2];
      passwordRAM_UINT8_6D[3] = passwordIn[3];
      passwordRAM_UINT8_6D[4] = passwordIn[4];
      passwordRAM_UINT8_6D[5] = passwordIn[5];
      passAssignedRAM_BOOL = passAssignedIn;
      gotoReady = true;
    (default) -> idle
    idle -> AssignPass [order 1] : [passSwitch==true]
    idle -> PassAssignedPreviously [order 2] : [passAssignedIn]
    AssignPass -> idle : [passSwitch==false]
  state closed
    entry:
    bulbPin_BOOL = false;
    leftMotor = CLOSED;
    rightMotor = CLOSED;
    openingActive = 0;
    gateState = CLOSED;
    closingTimer = 0;
    state openingGate
    state MonitorInput
      entry:
      passTimer = 0;
    state KpPassHandler
      du:
      passTimer++;
      state monitorBtnPressed
      state btnPressed
        entry:
        trialPass[counter] = KpCharPressed;
      state initTrailPass
        entry:
        initCounter = 1;
        state initiatePass
          entry:
          trialPass[initCounter] = 0;
        (junction 269) -> initiatePass
        (default) -> (junction 269)
        initiatePass -> (junction 269) : [initCounter < 5]...
            | /initCounter++;
      state verifyPass
        (default) -> (junction 115)
        (junction 115) -> (junction 116) [order 1] : [trialPass[0] != passwordRAM_UINT8_6D[0]]
        (junction 115) -> (junction 119) [order 2]
        (junction 116) -> (junction 118) : {passSuccess = WRONG_PASSWORD;}
        (junction 119) -> (junction 122) [order 1] : [trialPass[1] != passwordRAM_UINT8_6D[1]]
        (junction 119) -> (junction 120) [order 2]
        (junction 122) -> (junction 121) : {passSuccess = WRONG_PASSWORD;}
        (junction 120) -> (junction 144) [order 1] : [trialPass[2] != passwordRAM_UINT8_6D[2]]
        (junction 120) -> (junction 143) [order 2]
        (junction 144) -> (junction 168) : {passSuccess = WRONG_PASSWORD;}
        (junction 143) -> (junction 149) [order 1] : [trialPass[3] != passwordRAM_UINT8_6D[3]]
        (junction 143) -> (junction 153) [order 2]
        (junction 149) -> (junction 169) : {passSuccess = WRONG_PASSWORD;}
        (junction 153) -> (junction 156) [order 1] : [trialPass[4] != passwordRAM_UINT8_6D[4]]
        (junction 153) -> (junction 157) [order 2]
        (junction 156) -> (junction 170) : {passSuccess = WRONG_PASSWORD;}
        (junction 157) -> (junction 158) [order 1] : [trialPass[5] != passwordRAM_UINT8_6D[5]]
        (junction 157) -> (junction 164) [order 2] : {passSuccess = PASSWORD_VERIFIED;}
        (junction 158) -> (junction 171) : {passSuccess = WRONG_PASSWORD;}
        (junction 171) -> (junction 164)
        (junction 170) -> (junction 171)
        (junction 169) -> (junction 170)
        (junction 168) -> (junction 169)
        (junction 121) -> (junction 168)
        (junction 118) -> (junction 121)
        (junction 164) -> (junction 165)
      (default) -> initTrailPass
      monitorBtnPressed -> (junction 263) : [hasChanged...
          | (KpCharPressed)]
      (junction 263) -> btnPressed : [KpCharPressed != 0]/{counter++;}
      initTrailPass -> monitorBtnPressed : [initCounter == 5]...
          | /{counter = 0;}
      btnPressed -> monitorBtnPressed [order 1] : [counter < 5]
      (junction 262) -> initTrailPass : [(KpCharPressed == OPEN_CHAR)...
          |  && (KpCharPressed != 0)]...
          |  / {openingActive = OPENING_ACTIVE;}
      btnPressed -> verifyPass [order 2] : [counter >= 5]
      verifyPass -> (junction 262) : [hasChanged(KpCharPressed) && (passSuccess == PASSWORD_VERIFIED)]
    (default) -> MonitorInput
    MonitorInput -> openingGate [order 1] : [hasChanged(RFPressedOut_UINT8) && (RFPressedOut_UINT8 == true)]/{openingActive = OPENING_ACTIVE;}
    KpPassHandler -> MonitorInput [order 3] : [(passTimer == PASS_TIMEOUT)]
        | /passSuccess = TIMEOUT;
    KpPassHandler -> openingGate [order 1] : [openingActive == OPENING_ACTIVE]
    MonitorInput -> (junction 260) [order 2] : [hasChanged...
        | (KpCharPressed)]
    KpPassHandler -> MonitorInput [order 2] : [(passSuccess == WRONG_PASSWORD)]
    (junction 260) -> KpPassHandler : [(KpCharPressed != 0) ...
        | &&(KpCharPressed != OPEN_CHAR)...
        | &&(KpCharPressed != CLOSE_CHAR)...
        | && passAssignedRAM_BOOL...
        | && passSwitch == false]
        | /passSuccess = PASS_INCOMPLETE;...
        | trialPass[0] = KpCharPressed;
  state opening
    entry:
    bulbPin_BOOL = true;
    stableTimer = 0;
    gateState = OPENING;
    du:
    openingTimer++;
    state openLeftSide
      entry:
      leftMotor = OPENING;
      openSideDelay = 0;
      during:
      openSideDelay++;
    state openRightSide
      entry:
      rightMotor = OPENING;
      du:
      stableTimer += 1;
    (default) -> openLeftSide
    openLeftSide -> openRightSide : [openSideDelay == OPEN_SIDE_VALUE]
  state closing
    entry:
    gateState = CLOSING;
    du:
    closingTimer++;
    state closingRightSide
      entry:
      rightMotor = CLOSING;
      closeSideDelay = 0;
      during:
      closeSideDelay++;
    state closingLeftSide
      entry:
      leftMotor = CLOSING;
      du:
      stableTimer += 1;
    (default) -> closingRightSide
    closingRightSide -> closingLeftSide : [closeSideDelay == CLOSE_SIDE_VALUE]
  state open
    entry:
    gateState = OPEN;
    openingTimer = 0;
    state gateOpen
      entry:
      closing_active = false;
      leftMotor = OPEN;
      rightMotor = OPEN;
    state closing
      entry:
      closing_active = true;
    (default) -> gateOpen
    gateOpen -> open.closing [order 1] : [hasChanged(KpCharPressed) && (KpCharPressed == CLOSE_CHAR)]
    gateOpen -> open.closing [order 2] : [hasChanged(RFPressedOut_UINT8) && (RFPressedOut_UINT8 == true)]
  closed -> (junction 258) [order 1] : [hasChanged(passSwitch)]
  (junction 258) -> init : [passSwitch]
  (default) -> init
  closed -> opening [order 2] : [openingActive == OPENING_ACTIVE]
  init -> closed [order 1] : [gotoReady == true]
  init -> closed [order 2] : [hasChanged(RFPressedOut_UINT8)...
      | &&(RFPressedOut_UINT8 == true)]
  closing -> closed [order 1] : [(current_sensor == 0)...
      | &&(stableTimer >= STABLE_TIMER_VALUE)]...
      | /stableTimer = 0;
  closing -> closed [order 3] : [closingTimer >= MOVING_TIMER]
  closing -> closed [order 2] : [((hasChanged(RFPressedOut_UINT8)...
      | &&(RFPressedOut_UINT8 == true)) ...
      | || ((KpCharPressed == CLOSE_CHAR)...
      |  && hasChanged(KpCharPressed)))...
      | && (stableTimer >= STABLE_TIMER_VALUE)]...
      | /stableTimer = 0;
  opening -> open [order 2] : [((hasChanged(RFPressedOut_UINT8)...
      | &&(RFPressedOut_UINT8 == true)) ...
      | || ((KpCharPressed == OPEN_CHAR)...
      |  && hasChanged(KpCharPressed)))...
      | && (stableTimer >= STABLE_TIMER_VALUE)]...
      | /stableTimer = 0;
  opening -> open [order 3] : [openingTimer >= MOVING_TIMER]
  opening -> open [order 1] : [(current_sensor == 0)...
      | && (stableTimer >= STABLE_TIMER_VALUE)]...
      | /stableTimer = 0;
  open -> closing : [closing_active == true]
  data: KpCharPressed input; RFPressedOut_UINT8 input; openingActive local uint8; passSwitch input; trialPass local uint8 size=6; counter local uint8; closing_active local uint8; current_sensor input; initCounter local uint8; openSideDelay local uint16; leftMotor output uint8 =0; rightMotor output uint8 =0; bulbPin_BOOL output boolean; closeSideDelay local uint16; OPENING_ACTIVE input =2; WRONG_PASSWORD input =1; OPEN_SIDE_VALUE input =20; CLOSE_SIDE_VALUE input =20; PASSWORD_VERIFIED input =3; CLOSE_CHAR input =12; OPEN_CHAR input; OPENING input =2; CLOSED input =1; CLOSING input =4; OPEN input =3; passAssignedRAM_BOOL output boolean; gotoReady local boolean; passSuccess output uint8 =0; NO_PASS_ASSIG input; PASS_ASSIGNED input; PASS_INCOMPLETE input; PASS_TIMEOUT input; passTimer local uint16; TIMEOUT input; passwordRAM_UINT8_6D output uint8 size=6; passwordIn input size=6; passAssignedIn input; stableTimer local uint32; gateState output uint8; INIT input; closingTimer local uint32; openingTimer local uint32; MOVING_TIMER input; STABLE_TIMER_VALUE input

== stateflow chart GATE_B/CurrentFilterSubsystem/10msSmapler ==
  (default) -> (junction 2)
  (junction 2) -> (junction 3) : {counter_1ms++;}
  (junction 3) -> (junction 6) : [counter_1ms == 10]
      | {
      | triggerOn;
      | counter_1ms = 0;
      | }
  data: counter_1ms local double
  events: triggerOn output FUNCTION_CALL_EVENT

== stateflow chart GATE_B/CurrentFilterSubsystem/Subsystem/rightSquareWaveDetector ==
  state Running
    entry:
    counterHigh = 0;
    counterLow= 0;
    currentValue = 1;
    state High
      entry:
      counterLow = 0;
    state Low
      entry:
      counterHigh = 0;
    (default) -> High
    High -> High [order 2] : [CurrentAnalogIn > CURRENT_THRESH]
        | /counterHigh++;
    High -> Low [order 1] : [CurrentAnalogIn < CURRENT_THRESH]
    Low -> High [order 1] : [CurrentAnalogIn > CURRENT_THRESH]
    Low -> Low [order 2] : [CurrentAnalogIn < CURRENT_THRESH]
        | /counterLow++;
  state Stop
    entry:
    currentValue = 0;
    stableCounter = 0;
  (default) -> Stop
  Stop -> Running : [((CurrentAnalogInOld > CURRENT_THRESH)...
      |  && (CurrentAnalogIn < CURRENT_THRESH)) ...
      | || ((CurrentAnalogInOld < CURRENT_THRESH)...
      |  && (CurrentAnalogIn > CURRENT_THRESH))]
  Running -> Stop : [(counterHigh >= CURRENT_STABLE_TIMER)...
      |  || (counterLow >= CURRENT_STABLE_TIMER)]
  data: CurrentAnalogIn input; currentValue output uint8; counterHigh local uint16; counterLow local uint16; stableCounter local uint8; CurrentAnalogInOld input; CURRENT_STABLE_TIMER input; CURRENT_THRESH input
